simulink model "pt1_sin_waves_coulomb_viscous_friction"  (R2019a)
settings: Solver=ode4  StartTime=0.0  StopTime=1  FixedStep=0.001  RelTol=1e-3
libraries: simulink x3
settings Model: Creator=guima  LastModifiedBy=guima

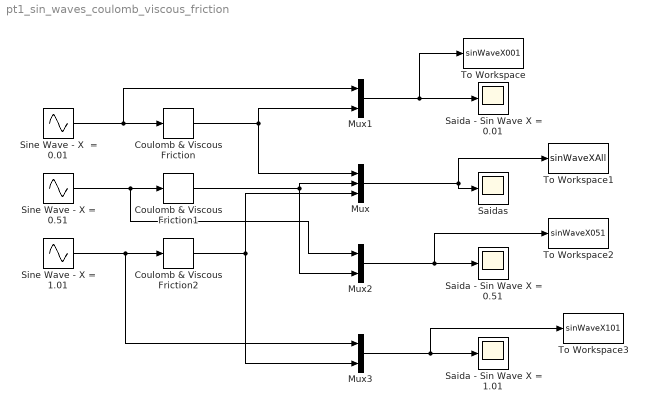
== system pt1_sin_waves_coulomb_viscous_friction ==
  Coulomb & Viscous Friction : simulink/Discontinuities/Coulomb & Viscous Friction  offset=0.1  gain=1
      settings: SourceProductName=Simulink
  Coulomb & Viscous Friction1 : simulink/Discontinuities/Coulomb & Viscous Friction  offset=0.1  gain=1
      settings: SourceProductName=Simulink
  Coulomb & Viscous Friction2 : simulink/Discontinuities/Coulomb & Viscous Friction  offset=0.1  gain=1
      settings: SourceProductName=Simulink
  Mux : Mux  Inputs=3
  Mux1 : Mux  Inputs=2
  Mux2 : Mux  Inputs=2
  Mux3 : Mux  Inputs=2
  Saida - Sin Wave X = 0.01 : Scope
  Saida - Sin Wave X = 0.51 : Scope
  Saida - Sin Wave X = 1.01 : Scope
  Saidas : Scope
  Sine Wave - X  = 0.01 : Sin  Amplitude=0.01  Frequency=2*pi  SampleTime=0
  Sine Wave - X = 0.51 : Sin  Amplitude=0.51  Frequency=2*pi  SampleTime=0
  Sine Wave - X = 1.01 : Sin  Amplitude=1.01  Frequency=2*pi  SampleTime=0
  To Workspace : ToWorkspace  VariableName=sinWaveX001  SaveFormat=Structure With Time  SampleTime=-1
  To Workspace1 : ToWorkspace  VariableName=sinWaveXAll  SaveFormat=Structure With Time  SampleTime=-1
  To Workspace2 : ToWorkspace  VariableName=sinWaveX051  SaveFormat=Structure With Time  SampleTime=-1
  To Workspace3 : ToWorkspace  VariableName=sinWaveX101  SaveFormat=Structure With Time  SampleTime=-1
  wires:
  Coulomb & Viscous Friction1/1 -> Mux2/2, Mux/2
  Sine Wave - X = 0.51/1 -> Coulomb & Viscous Friction1/1, Mux2/1
  Sine Wave - X  = 0.01/1 -> Coulomb & Viscous Friction/1, Mux1/1
  Mux1/1 -> To Workspace/1, Saida - Sin Wave X = 0.01/1
  Mux3/1 -> To Workspace3/1, Saida - Sin Wave X = 1.01/1
  Coulomb & Viscous Friction/1 -> Mux/1, Mux1/2
  Mux2/1 -> To Workspace2/1, Saida - Sin Wave X = 0.51/1
  Mux/1 -> Saidas/1, To Workspace1/1
  Coulomb & Viscous Friction2/1 -> Mux3/2, Mux/3
  Sine Wave - X = 1.01/1 -> Coulomb & Viscous Friction2/1, Mux3/1
